simulink model "calculate_troom_transfer"  (R2016b)
settings: Solver=ode45  StartTime=0.0  StopTime=24*3600  RelTol=1e-3
settings Model: Creator=drhf  LastModifiedBy=drhf
settings DataIOCC: ReturnWorkspaceOutputs=on
settings DebuggingCC: ReadBeforeWriteMsg=DisableAll  WriteAfterWriteMsg=DisableAll  WriteAfterReadMsg=DisableAll  MultiTaskDSMMsg=none
settings ModelReferenceCC: UpdateModelReferenceTargets=IfOutOfDate
settings SFSimCC: SFSimEcho=off

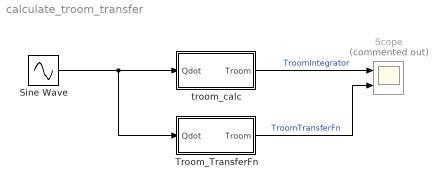
== system calculate_troom_transfer ==
  Scope : Scope  Commented=on  NumInputPorts=2
  Sine Wave : Sin  Amplitude=1000  Frequency=2*pi/24/3600  SampleTime=0
  Troom_TransferFn : Subsystem  mask(Calculate room temperature){A=140, capa=0.5e6, Denominator=[70000000 0], tini=20, dtroom=inf}
      mask prompts: A "Heated surface of the house in m²"; capa "Thermal capactiy per surface in J/m²/K"; tini "Initial temperature in °C"; dtroom "Max. change of room temperature in K"
      mask help:
      | One node thermal model based on energy balance.
      | The room temperature can be limited by "Max. change of room temperature" . The temperature is limited by this parameter, the result of the energy balance (Qdot_all) is the required power to maintain the limit.
      mask init:
      | Cap = max(1,capa*A);
      | de = ['[', num2str(Cap), ' 0]'];
      | set_param(gcb,'Denominator', de);
      mask TypeOptions Denominator: Transfer Fcn/Denominator
      mask TypeOptions tini: Tini/Value | add_Tini/Bias
      mask DialogControl Container3 Prompt: Transfer function coefficients from thermal capacity
  troom_calc : Subsystem  mask(Calculate room temperature){A=140, capa=0.5e6, tini=20, dtroom=inf}
      mask prompts: A "Heated surface of the house in m²"; capa "Thermal capactiy per surface in J/m²/K"; tini "Initial temperature in °C"; dtroom "Max. change of room temperature in K"
      mask help:
      | One node thermal model based on energy balance.
      | The room temperature can be limited by "Max. change of room temperature" . The temperature is limited by this parameter, the result of the energy balance (Qdot_all) is the required power to maintain the limit.
      mask TypeOptions A: A/Value
      mask TypeOptions capa: capa/Value
      mask TypeOptions tini: Tini/Value | add_Tini/Bias
  wires:
  Sine Wave/1 -> Troom_TransferFn/1(Qdot), troom_calc/1(Qdot)
  troom_calc/1(Troom) -> Scope/1  "TroomIntegrator"
  Troom_TransferFn/1(Troom) -> Scope/2  "TroomTransferFn"

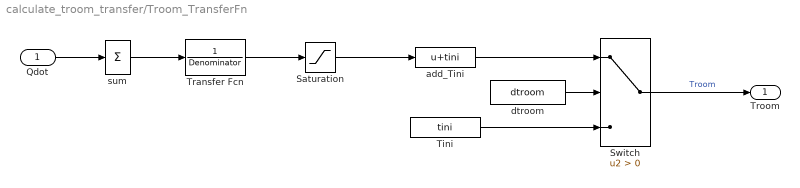
== system calculate_troom_transfer/Troom_TransferFn ==
  Qdot : Inport
  Saturation : Saturate  UpperLimit=dtroom  LowerLimit=-dtroom
  Switch : Switch  Criteria=u2 > Threshold
  Tini : Constant  Value=tini
  Transfer Fcn : TransferFcn  Denominator=Denominator
  add_Tini : Bias  Bias=tini
  dtroom : Constant  Value=dtroom
  sum : Sum  Inputs=1  SaturateOnIntegerOverflow=on  InputSameDT=on  OutDataTypeStr=Inherit: Same as first input
  Troom : Outport
  wires:
  add_Tini/1 -> Switch/1
  dtroom/1 -> Switch/2
  Tini/1 -> Switch/3
  Qdot/1 -> sum/1
  Switch/1 -> Troom/1  "Troom"
  Transfer Fcn/1 -> Saturation/1
  sum/1 -> Transfer Fcn/1
  Saturation/1 -> add_Tini/1

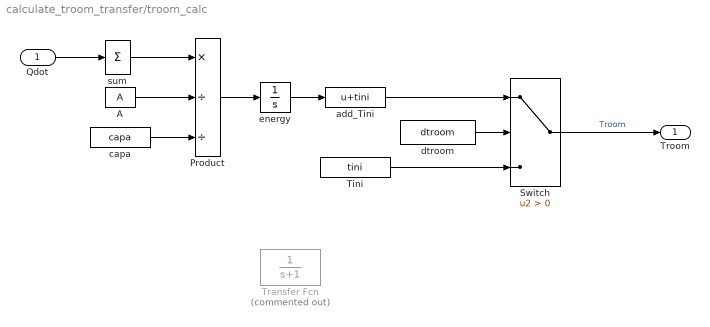
== system calculate_troom_transfer/troom_calc ==
  Qdot : Inport
  A : Constant  Value=A
  Product : Product  Inputs=*//
  Switch : Switch  Criteria=u2 > Threshold
  Tini : Constant  Value=tini
  Transfer Fcn : TransferFcn  Commented=on  Denominator=[1 1]
  add_Tini : Bias  Bias=tini
  capa : Constant  Value=capa
  dtroom : Constant  Value=dtroom
  energy : Integrator  LimitOutput=on  UpperSaturationLimit=dtroom  LowerSaturationLimit=min(-dtroom, -0.01)
  sum : Sum  Inputs=1  SaturateOnIntegerOverflow=on  InputSameDT=on  OutDataTypeStr=Inherit: Same as first input
  Troom : Outport
  wires:
  sum/1 -> Product/1
  Product/1 -> energy/1
  energy/1 -> add_Tini/1
  Switch/1 -> Troom/1  "Troom"
  Qdot/1 -> sum/1
  A/1 -> Product/2
  capa/1 -> Product/3
  Tini/1 -> Switch/3
  dtroom/1 -> Switch/2
  add_Tini/1 -> Switch/1
